simulink model "JC_20220328_1432"  (R2021a)
settings: Solver=FixedStepAuto  StartTime=0.0  StopTime=inf  FixedStep=1e-3  RelTol=1e-3  EnableMultiTasking=on
values from neighbouring files (symbols this model uses):
  a = 1.43208    [1DoFRollParam.mat]
  b = 1.62792    [1DoFRollParam.mat]    (also in cmenv_20220308_0532.m = ~isempty(strfind(computer, '64')))
  Cq = 8888.064375    [1DoFRollParam.mat]
  FzF_0_w = 6523.65    [1DoFRollParam.mat]
  FzR_0_w = 5738.85    [1DoFRollParam.mat]
  h_CoG = 0.642    [1DoFRollParam.mat]
  h_RC = 0.116    [1DoFRollParam.mat]
  hs = 0.526    [1DoFRollParam.mat]
  hu = 0.4    [1DoFRollParam.mat]
  Ix = 850    [1DoFRollParam.mat]
  Iz = 4600    [1DoFRollParam.mat]
  Kq = 138929.062472    [1DoFRollParam.mat]
  M = 2500    [1DoFRollParam.mat]
  M_damp_f = [-2800.47 -2055.7 -1627.71 -1221.625 -703.4875 0 703.4875 1221.625 1627.71 2055.7 2800.47]    [1DoFRollParam.mat]
  M_damp_r = [-2742.3 -2013 -1593.9 -1196.25 -688.875 0 688.875 1196.25 1593.9 2013 2742.3]    [1DoFRollParam.mat]
  Mf_stiff = [-6881.2026603 -6818.65169539 -6756.10058191 -6693.54932121 -6630.99791467 -6568.44636364 -6505.89466949 -6443.34283357 -6380.79085727 -6318.23874192 -6255.68648891 -6193.13409959 ... (221 elements, 1x221)]    [1DoFRollParam.mat]    (also in roll_stiffness.mat)
  Mr_stiff = [-8903.36440298 -8822.14706815 -8740.93733551 -8659.73513552 -8578.54039868 -8497.35305544 -8416.17303626 -8335.00027161 -8253.83469192 -8172.67622765 -8091.52480923 -8010.38036709 ... (221 elements, 1x221)]    [1DoFRollParam.mat]    (also in roll_stiffness.mat)
  ms = 2159    [1DoFRollParam.mat]
  mu = 341    [1DoFRollParam.mat]
  theta_dot_f_damp = [-0.617210682493 -0.308605341246 -0.154302670623 -0.0593471810089 -0.0237388724036 0 0.0237388724036 0.0593471810089 0.154302670623 0.308605341246 0.617210682493]    [1DoFRollParam.mat]
  theta_dot_r_damp = [-0.630303030303 -0.315151515152 -0.157575757576 -0.0606060606061 -0.0242424242424 0 0.0242424242424 0.0606060606061 0.157575757576 0.315151515152 0.630303030303]    [1DoFRollParam.mat]
  theta_f_stiff = [-0.13056379822 -0.129376854599 -0.128189910979 -0.127002967359 -0.125816023739 -0.124629080119 -0.123442136499 -0.122255192878 -0.121068249258 -0.119881305638 -0.118694362018 -0.117507418398 ... (221 elements, 1x221)]    [1DoFRollParam.mat]    (also in roll_stiffness.mat)
  theta_r_stiff = [-0.133333333333 -0.132121212121 -0.130909090909 -0.129696969697 -0.128484848485 -0.127272727273 -0.126060606061 -0.124848484848 -0.123636363636 -0.122424242424 -0.121212121212 -0.12 ... (221 elements, 1x221)]    [1DoFRollParam.mat]    (also in roll_stiffness.mat)
  tw = 1.6675    [1DoFRollParam.mat]
undefined symbols (not defined in the file or in its folder): Continuous, DiscIntNeverNeededParam, params, Time, X0
libraries: CarMaker4SL x52, simulink x2, ctrlSharedLib x2
(part 3 of 3)

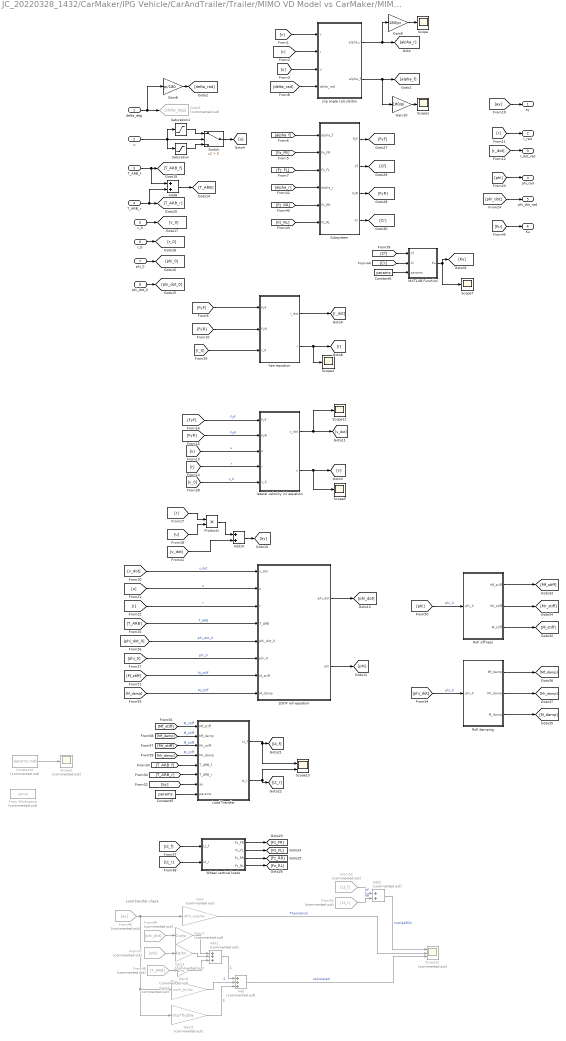
== system JC_20220328_1432/CarMaker/IPG Vehicle/CarAndTrailer/Trailer/MIMO VD Model vs CarMaker/MIMO 1DOF roll with LT1 ==
  note: Load transfer check
  delta_deg : Inport
  u : Inport  Port=2
  T_ARB_f : Inport  Port=3
  T_ARB_r : Inport  Port=4
  v_0 : Inport  Port=5
  r_0 : Inport  Port=6
  phi_0 : Inport  Port=7
  phi_dot_0 : Inport  Port=8
  1DOF roll equation : Subsystem
  Add : Sum  Commented=on  Inputs=+++
  Add1 : Sum  Commented=on  Inputs=+++
  Add10 : Sum
  Add2 : Sum  Commented=on
  Add8 : Sum
  Constant4 : Constant  Commented=on  Value=params.mat
  Constant5 : Constant  Value=params
  Constant6 : Constant  Value=params
  From Workspace : FromWorkspace  Commented=on  VariableName=simin
  From46 : From  Commented=on  GotoTag=ay
  From47 : From  Commented=on  GotoTag=phi
  From48 : From  Commented=on  GotoTag=T_ARB
  From49 : From  Commented=on  GotoTag=phi_dot
  From52 : From  Commented=on  GotoTag=Lt_f
  From53 : From  Commented=on  GotoTag=Lt_r
  Gain : Gain  Commented=on  Gain=M*h_CoG/tw
  Gain1 : Gain  Commented=on  Gain=Kq/tw
  Gain10 : Gain  Gain=180/pi
  Gain4 : Gain  Commented=on  Gain=ms*h_RC/tw
  Gain5 : Gain  Commented=on  Gain=mu*hu/tw
  Gain6 : Gain  Commented=on  Gain=1/tw
  Gain7 : Gain  Commented=on  Gain=Cq/tw
  Gain8 : Gain  Gain=pi/180
  Gain9 : Gain  Gain=180/pi
  Goto5 : Goto  Commented=on  GotoTag=delta_deg
  Load Transfer : MATLAB Function  TreatAsAtomicUnit=on
  MATLAB Function : MATLAB Function  TreatAsAtomicUnit=on
  Product1 : Product
  Roll damping : Subsystem
  Roll siffness : Subsystem
  Saturation : Saturate  UpperLimit=-eps  LowerLimit=-inf
  Saturation1 : Saturate  UpperLimit=inf  LowerLimit=eps
  Scope{,1,4..5,7,11} (6 alike) : Scope
  Scope12 : Scope  Commented=on  NumInputPorts=3
  Scope13 : Scope  NumInputPorts=2
  Scope2 : Scope  Commented=on
  Subsystem : Subsystem
      settings: AttributesFormatString=%<MinAlgLoopOccurrences>
  Switch : Switch  Criteria=u2 > Threshold
  Wheel vertical loads : Subsystem
      settings: AttributesFormatString=%<MinAlgLoopOccurrences>
  Yaw equation : Subsystem
  lateral velocity (v) equation : Subsystem
  slip angle calculaiton : Subsystem
  ay : Outport
  r_rad : Outport  Port=2
  r_dot_rad : Outport  Port=3
  phi_rad : Outport  Port=4
  phi_dot_rad : Outport  Port=5
  Ku : Outport  Port=6
  wires:
  delta_deg/1 -> Gain8/1, Goto5/1
  [r] -> r_rad/1
  [r_dot] -> r_dot_rad/1
  [r] -> Product1/1
  [u] -> Product1/2
  [ay] -> ay/1
  Gain8/1 -> [delta_rad]
  Gain10/1 -> Scope1/1
  Gain9/1 -> Scope/1
  [phi] -> phi_rad/1
  [phi_dot] -> phi_dot_rad/1
  phi_dot_0/1 -> [phi_dot_0]
  T_ARB_f/1 -> Add8/1, [T_ARB_f]
  T_ARB_r/1 -> Add8/2, [T_ARB_r]
  Add8/1 -> [T_ARB]
  [T_ARB_r] -> Load Transfer/6(T_ARB_r)
  [T_ARB_f] -> Load Transfer/5(T_ARB_f)
  Load Transfer/1(Lt_f) -> Scope13/1, [Lt_f]
  Load Transfer/2(Lt_r) -> Scope13/2, [Lt_r]
  Add10/1 -> [ay]
  Product1/1 -> Add10/1
  [v_dot] -> Add10/2
  [ay] -> Load Transfer/7(ay)
  [Lt_r] -> Wheel vertical loads/2(Lt_r)
  [Lt_f] -> Wheel vertical loads/1(Lt_f)
  Wheel vertical loads/1(Fz_FR) -> [Fz_FR]
  Wheel vertical loads/2(Fz_FL) -> [Fz_FL]
  Wheel vertical loads/3(Fz_RR) -> [Fz_RR]
  Wheel vertical loads/4(Fz_RL) -> [Fz_RL]
  slip angle calculaiton/2(alpha_f) -> Gain10/1, [alpha_f]
  slip angle calculaiton/1(alpha_r) -> [alpha_r], Gain9/1
  [v] -> slip angle calculaiton/1(v)
  [r] -> slip angle calculaiton/2(r)
  [u] -> slip angle calculaiton/3(u)
  [delta_rad] -> slip angle calculaiton/4(delta_rad)
  [alpha_f] -> Subsystem/1(alpha_f)
  [Fz_FR] -> Subsystem/2(Fz_FR)
  [Fz_FL] -> Subsystem/3(Fz_FL)
  [alpha_r] -> Subsystem/4(alpha_r)
  [Fz_RR] -> Subsystem/5(Fz_RR)
  [Fz_RL] -> Subsystem/6(Fz_RL)
  Subsystem/1(FyF) -> [FyF]
  Subsystem/3(FyR) -> [FyR]
  [Cr] -> MATLAB Function/2(Cr)
  [Cf] -> MATLAB Function/1(Cf)
  MATLAB Function/1(Ku) -> Scope7/1, [Ku]
  [Ku] -> Ku/1
  Subsystem/4(Cr) -> [Cr]
  Subsystem/2(Cf) -> [Cf]
  Yaw equation/2(r) -> [r], Scope4/1
  [FyF] -> Yaw equation/1(FyF)
  [FyR] -> Yaw equation/2(FyR)
  [r_0] -> Yaw equation/3(r_0)
  Yaw equation/1(r_dot) -> [r_dot]
  lateral velocity (v) equation/2(v) -> [v], Scope5/1
  lateral velocity (v) equation/1(v_dot) -> [v_dot], Scope11/1
  [FyF] -> lateral velocity (v) equation/1(FyF)  "FyF"
  [FyR] -> lateral velocity (v) equation/2(FyR)  "FyR"
  [u] -> lateral velocity (v) equation/3(u)  "u"
  [r] -> lateral velocity (v) equation/4(r)  "r"
  [v_0] -> lateral velocity (v) equation/5(v_0)  "v_0"
  [v_dot] -> 1DOF roll equation/1(v_dot)  "v_dot"
  [u] -> 1DOF roll equation/2(u)  "u"
  [r] -> 1DOF roll equation/3(r)  "r"
  [T_ARB] -> 1DOF roll equation/4(T_ARB)  "T_ARB"
  [phi_dot_0] -> 1DOF roll equation/5(phi_dot_0)  "phi_dot_0"
  [phi_0] -> 1DOF roll equation/6(phi_0)  "phi_0"
  1DOF roll equation/1(phi_dot) -> [phi_dot]
  1DOF roll equation/2(phi) -> [phi]
  phi_0/1 -> [phi_0]
  r_0/1 -> [r_0]
  v_0/1 -> [v_0]
  From46/1 -> Gain5/1, Gain4/1, Gain/1
  Gain/1 -> Scope12/2  "Theoretical"
  From47/1 -> Gain1/1
  Gain4/1 -> Add/2  "2"
  Gain5/1 -> Add/3  "3"
  Add/1 -> Scope12/3  "calculated"
  Gain1/1 -> Add1/2
  Add1/1 -> Add/1  "1"
  From48/1 -> Gain6/1
  Gain6/1 -> Add1/3
  From49/1 -> Gain7/1
  Gain7/1 -> Add1/1
  Add2/1 -> Scope12/1  "matlabFCN"
  From53/1 -> Add2/2  "ltR"
  From52/1 -> Add2/1  "ltF"
  [phi] -> Roll siffness/1(phi_0)  "phi_0"
  Roll siffness/1(Mf_stiff) -> [Mf_stiff]
  Roll siffness/3(M_stiff) -> [M_stiff]
  Roll siffness/2(Mr_stiff) -> [Mr_stiff]
  [M_stiff] -> 1DOF roll equation/7(M_stiff)  "M_stiff"
  Roll damping/3(M_damp) -> [M_damp]
  Roll damping/1(Mf_damp) -> [Mf_damp]
  Roll damping/2(Mr_damp) -> [Mr_damp]
  [phi_dot] -> Roll damping/1(phi_0)  "phi_0"
  [M_damp] -> 1DOF roll equation/8(M_damp)  "M_stiff"
  [Mf_stiff] -> Load Transfer/1(Mf_stiff)  "M_stiff"
  [Mf_damp] -> Load Transfer/2(Mf_damp)  "M_stiff"
  [Mr_stiff] -> Load Transfer/3(Mr_stiff)  "M_stiff"
  [Mr_damp] -> Load Transfer/4(Mr_damp)  "M_stiff"
  Constant4/1 -> Scope2/1
  Constant5/1 -> Load Transfer/8(params)
  Constant6/1 -> MATLAB Function/3(params)
  Saturation1/1 -> Switch/1
  u/1 -> Saturation/1, Saturation1/1, Switch/2
  Saturation/1 -> Switch/3
  Switch/1 -> [u]

== system JC_20220328_1432/CarMaker/IPG Vehicle/CarAndTrailer/Trailer/MIMO VD Model vs CarMaker/MIMO 1DOF roll with LT1/1DOF roll equation ==
  v_dot : Inport
  u : Inport  Port=2
  r : Inport  Port=3
  T_ARB : Inport  Port=4
  phi_dot_0 : Inport  Port=5
  phi_0 : Inport  Port=6
  M_stiff : Inport  Port=7
  M_damp : Inport  Port=8
  Add6 : Sum
  Add7 : Sum  Inputs=+---
  Gain11 : Gain  Gain=1/Ix
  Gain12 : Gain  Gain=ms*hs
  Integrator2 : Integrator  InitialConditionSource=external
  Integrator3 : Integrator  InitialConditionSource=external
  Product2 : Product
  phi_dot : Outport
  phi : Outport  Port=2
  wires:
  Gain11/1 -> Integrator2/1  "phi_dot_dot"
  Integrator3/1 -> phi/1  "phi"
  Integrator2/1 -> phi_dot/1, Integrator3/1  "phi_dot"
  Add7/1 -> Gain11/1
  Add6/1 -> Gain12/1
  Product2/1 -> Add6/2
  Gain12/1 -> Add7/1
  phi_0/1 -> Integrator3/2
  v_dot/1 -> Add6/1
  phi_dot_0/1 -> Integrator2/2
  T_ARB/1 -> Add7/4
  u/1 -> Product2/1
  r/1 -> Product2/2
  M_stiff/1 -> Add7/2
  M_damp/1 -> Add7/3

== system JC_20220328_1432/CarMaker/IPG Vehicle/CarAndTrailer/Trailer/MIMO VD Model vs CarMaker/MIMO 1DOF roll with LT1/Roll damping ==
  phi_0 : Inport
  Add3 : Sum
  Front roll damping : Lookup_n-D  NumberOfTableDimensions=1  BreakpointsForDimension1=theta_dot_f_damp  Table=M_damp_f  InternalRulePriority=Speed  RndMeth=Simplest  InputSameDT=on
  Rear roll damping : Lookup_n-D  NumberOfTableDimensions=1  BreakpointsForDimension1=theta_dot_r_damp  Table=M_damp_r  InternalRulePriority=Speed  RndMeth=Simplest  InputSameDT=on
  Mf_damp : Outport
  Mr_damp : Outport  Port=2
  M_damp : Outport  Port=3
  wires:
  Front roll damping/1 -> Mf_damp/1, Add3/1
  phi_0/1 -> Rear roll damping/1, Front roll damping/1
  Rear roll damping/1 -> Mr_damp/1, Add3/2
  Add3/1 -> M_damp/1

== system JC_20220328_1432/CarMaker/IPG Vehicle/CarAndTrailer/Trailer/MIMO VD Model vs CarMaker/MIMO 1DOF roll with LT1/Roll siffness ==
  phi_0 : Inport
  Add3 : Sum
  Front roll stiffness : Lookup_n-D  NumberOfTableDimensions=1  BreakpointsForDimension1=theta_f_stiff  Table=Mf_stiff  InternalRulePriority=Speed  RndMeth=Simplest  InputSameDT=on
  Rear roll stiffness : Lookup_n-D  NumberOfTableDimensions=1  BreakpointsForDimension1=theta_r_stiff  Table=Mr_stiff  InternalRulePriority=Speed  RndMeth=Simplest  InputSameDT=on
  Mf_stiff : Outport
  Mr_stiff : Outport  Port=2
  M_stiff : Outport  Port=3
  wires:
  Front roll stiffness/1 -> Mf_stiff/1, Add3/1
  phi_0/1 -> Rear roll stiffness/1, Front roll stiffness/1
  Rear roll stiffness/1 -> Mr_stiff/1, Add3/2
  Add3/1 -> M_stiff/1

== system JC_20220328_1432/CarMaker/IPG Vehicle/CarAndTrailer/Trailer/MIMO VD Model vs CarMaker/MIMO 1DOF roll with LT1/Subsystem ==
  alpha_f : Inport
  Fz_FR : Inport  Port=2
  Fz_FL : Inport  Port=3
  alpha_r : Inport  Port=4
  Fz_RR : Inport  Port=5
  Fz_RL : Inport  Port=6
  Add{,1..3} (4 alike) : Sum
  Front tire formula : MATLAB Function  TreatAsAtomicUnit=on
      settings: AttributesFormatString=%<MinAlgLoopOccurrences>  MinAlgLoopOccurrences=on
  Front tire formula1 : MATLAB Function  TreatAsAtomicUnit=on
      settings: MinAlgLoopOccurrences=on
  Rear tire formula : MATLAB Function  TreatAsAtomicUnit=on
      settings: MinAlgLoopOccurrences=on
  Rear tire formula1 : MATLAB Function  TreatAsAtomicUnit=on
      settings: MinAlgLoopOccurrences=on
  Scope1 : Scope  NumInputPorts=2
  FyF : Outport
  Cf : Outport  Port=2
  FyR : Outport  Port=3
  Cr : Outport  Port=4
  wires:
  Rear tire formula/1(Fy) -> Add1/1  "FyRR"
  Fz_RL/1 -> Rear tire formula1/2(Fz)
  Fz_RR/1 -> Rear tire formula/2(Fz)
  Rear tire formula1/1(Fy) -> Add1/2  "FyRL"
  Fz_FR/1 -> Front tire formula/2(Fz)
  Fz_FL/1 -> Front tire formula1/2(Fz)
  alpha_f/1 -> Front tire formula1/1(alpha_f), Front tire formula/1(alpha_f)
  alpha_r/1 -> Rear tire formula1/1(alpha_r), Rear tire formula/1(alpha_r)
  Front tire formula/1(Fy) -> Scope1/1, Add/1  "FyFR"
  Front tire formula1/1(Fy) -> Scope1/2, Add/2  "FYFL"
  Add/1 -> FyF/1
  Add1/1 -> FyR/1
  Front tire formula/2(C_f) -> Add2/1
  Front tire formula1/2(C_f) -> Add2/2
  Add2/1 -> Cf/1
  Rear tire formula/2(C_r) -> Add3/1
  Rear tire formula1/2(C_r) -> Add3/2
  Add3/1 -> Cr/1

== system JC_20220328_1432/CarMaker/IPG Vehicle/CarAndTrailer/Trailer/MIMO VD Model vs CarMaker/MIMO 1DOF roll with LT1/Wheel vertical loads ==
  Lt_f : Inport
  Lt_r : Inport  Port=2
  Constant : Constant  Value=FzF_0_w
  Constant1 : Constant  Value=FzR_0_w
  Sum : Sum  Inputs=|++
  Sum1 : Sum  Inputs=|++
  Sum2 : Sum  Inputs=+-|
  Sum3 : Sum  Inputs=+-|
  Fz_FR : Outport
  Fz_FL : Outport  Port=2
  Fz_RR : Outport  Port=3
  Fz_RL : Outport  Port=4
  wires:
  Constant/1 -> Sum2/1, Sum/1
  Constant1/1 -> Sum1/1, Sum3/1
  Sum1/1 -> Fz_RR/1
  Lt_f/1 -> Sum/2, Sum2/2
  Sum/1 -> Fz_FR/1
  Sum2/1 -> Fz_FL/1
  Lt_r/1 -> Sum1/2, Sum3/2
  Sum3/1 -> Fz_RL/1

== system JC_20220328_1432/CarMaker/IPG Vehicle/CarAndTrailer/Trailer/MIMO VD Model vs CarMaker/MIMO 1DOF roll with LT1/Yaw equation ==
  FyF : Inport
  FyR : Inport  Port=2
  r_0 : Inport  Port=3
  Add3 : Sum  Inputs=+-
  Gain4 : Gain  Gain=1/Iz
  Gain5 : Gain  Gain=a
  Gain6 : Gain  Gain=b
  Integrator : Integrator  InitialConditionSource=external
  r_dot : Outport
  r : Outport  Port=2
  wires:
  Gain4/1 -> r_dot/1, Integrator/1  "r_dot"
  FyF/1 -> Gain5/1
  r_0/1 -> Integrator/2
  Gain5/1 -> Add3/1
  Gain6/1 -> Add3/2
  Add3/1 -> Gain4/1
  FyR/1 -> Gain6/1
  Integrator/1 -> r/1  "r"

== system JC_20220328_1432/CarMaker/IPG Vehicle/CarAndTrailer/Trailer/MIMO VD Model vs CarMaker/MIMO 1DOF roll with LT1/lateral velocity (v) equation ==
  FyF : Inport
  FyR : Inport  Port=2
  u : Inport  Port=3
  r : Inport  Port=4
  v_0 : Inport  Port=5
  Add4 : Sum  Inputs=+-
  Add5 : Sum
  Gain7 : Gain  Gain=1/M
  Integrator1 : Integrator  InitialConditionSource=external
  Product : Product
  v_dot : Outport
  v : Outport  Port=2
  wires:
  Add4/1 -> v_dot/1, Integrator1/1  "v_dot"
  FyF/1 -> Add5/1
  Product/1 -> Add4/2
  Gain7/1 -> Add4/1
  Add5/1 -> Gain7/1
  Integrator1/1 -> v/1  "v"
  r/1 -> Product/2
  u/1 -> Product/1
  FyR/1 -> Add5/2
  v_0/1 -> Integrator1/2

== system JC_20220328_1432/CarMaker/IPG Vehicle/CarAndTrailer/Trailer/MIMO VD Model vs CarMaker/MIMO 1DOF roll with LT1/slip angle calculaiton ==
  v : Inport
  r : Inport  Port=2
  u : Inport  Port=3
  delta_rad : Inport  Port=4
  Add : Sum  Inputs=-+
  Add1 : Sum
  Add2 : Sum  Inputs=+-
  Divide : Product  Inputs=*/
  Divide1 : Product  Inputs=*/
  Gain : Gain  Gain=b
  Gain1 : Gain  Gain=a
  alpha_r : Outport
  alpha_f : Outport  Port=2
  wires:
  Gain1/1 -> Add1/2
  Divide1/1 -> Add2/2
  Add/1 -> Divide/1
  Add1/1 -> Divide1/1
  delta_rad/1 -> Add2/1
  r/1 -> Gain1/1, Gain/1
  Gain/1 -> Add/2
  Add2/1 -> alpha_f/1
  v/1 -> Add1/1, Add/1
  Divide/1 -> alpha_r/1
  u/1 -> Divide1/2, Divide/2

== matlab function JC_20220328_1432/CarMaker/IPG Vehicle/CarAndTrailer/Trailer/MIMO VD Model vs CarMaker/MIMO 1DOF roll with LT1/Load Transfer ==
  data: Mf_stiff input; Mf_damp input; Mr_stiff input; Mr_damp input; Lt_f output; Lt_r output; T_ARB_f input; T_ARB_r input; ay input; params input
function [Lt_f, Lt_r] = fcn(Mf_stiff, Mf_damp, Mr_stiff, Mr_damp, T_ARB_f, T_ARB_r, ay, params)

mu_f = params(1);
mu_r = params(2);
ms_f = params(3);
ms_r = params(4);
hu = params(5);
h_RC = params(6);
tw_F = params(7);
tw_R = params(8);

% St = load('params.mat');
% St2 = load('params2.mat');


%% Load transfer in the front
Ltf_1 = (Mf_stiff + Mf_damp + T_ARB_f)/tw_F; %% Load transfer due to roll (front)
Ltf_2 = ms_f*ay*h_RC/tw_F;
Ltf_3 = mu_f*ay*hu/tw_F;

Lt_f = Ltf_1 + Ltf_2 + Ltf_3;

%% Load transfer in the rear
Ltr_1 = (Mr_stiff + Mr_damp + T_ARB_r)/tw_R; %% Load transfer due to roll (front)
Ltr_2 = ms_r*ay*h_RC/tw_R;
Ltr_3 = mu_r*ay*hu/tw_R;

Lt_r = Ltr_1 + Ltr_2 + Ltr_3;

== matlab function JC_20220328_1432/CarMaker/IPG Vehicle/CarAndTrailer/Trailer/MIMO VD Model vs CarMaker/MIMO 1DOF roll with LT1/MATLAB Function ==
  data: Cf input; Ku output; Cr input; params input
function Ku = fcn(Cf, Cr, params)

a = params(9);
b = params(10);
M = params(11);
L = params(12);


Ku = M/L*((b*Cr - a*Cf)/(Cf*Cr));

== matlab function JC_20220328_1432/CarMaker/IPG Vehicle/CarAndTrailer/Trailer/MIMO VD Model vs CarMaker/MIMO 1DOF roll with LT1/Subsystem/Front tire formula ==
  data: alpha_f input; Fy output; Fz input; C_f output
function [Fy, C_f] = fcn(alpha_f, Fz)
%% Pajecka formula for the front axle

mu_peak = 1.37 - Fz*0.026/1000;
mu_90_deg_f = 0.723*mu_peak;

Bf = 13; %% stiffness factor. Gives maximum mu for alpha = 6º for the static front tyre load.
Cf = 1.515; % Makes mu_max/mu_90_deg=0.723 for static front tyre load
Df = mu_peak; %% peak value. If Df<Dr understeer
Ef = Fz*(0.5+2)/12000 - 2; %% Curvature factor. Linear variation from Fz = 0KN to 12KN

mu_y_f = Df.*sin(Cf.*atan(Bf*alpha_f - Ef*(Bf*alpha_f - atan(Bf*alpha_f))));

n_f = (Cf.*Df.*cos(Cf.*atan(Bf.*alpha_f + Ef.*(atan(Bf.*alpha_f) - Bf.*alpha_f))).*(Bf - Ef.*(Bf - Bf./(Bf.^2.*alpha_f.^2 + 1))))./((Bf.*alpha_f + Ef.*(atan(Bf.*alpha_f) - Bf.*alpha_f)).^2 + 1);
C_f = n_f.*Fz;

Fy = mu_y_f*Fz;

% Fy = alpha;

== matlab function JC_20220328_1432/CarMaker/IPG Vehicle/CarAndTrailer/Trailer/MIMO VD Model vs CarMaker/MIMO 1DOF roll with LT1/Subsystem/Front tire formula1 ==
  data: alpha_f input; Fy output; Fz input; C_f output
function [Fy, C_f] = fcn(alpha_f, Fz)
%% Pajecka formula for the front axle

mu_peak = 1.37 - Fz*0.026/1000;
mu_90_deg_f = 0.723*mu_peak;

Bf = 13; %% stiffness factor. Gives maximum mu for alpha = 6º for the static front tyre load.
Cf = 1.515; % Makes mu_max/mu_90_deg=0.723 for static front tyre load
Df = mu_peak; %% peak value. If Df<Dr understeer
Ef = Fz*(0.5+2)/12000 - 2; %% Curvature factor. Linear variation from Fz = 0KN to 12KN

mu_y_f = Df.*sin(Cf.*atan(Bf*alpha_f - Ef*(Bf*alpha_f - atan(Bf*alpha_f))));

n_f = (Cf.*Df.*cos(Cf.*atan(Bf.*alpha_f + Ef.*(atan(Bf.*alpha_f) - Bf.*alpha_f))).*(Bf - Ef.*(Bf - Bf./(Bf.^2.*alpha_f.^2 + 1))))./((Bf.*alpha_f + Ef.*(atan(Bf.*alpha_f) - Bf.*alpha_f)).^2 + 1);
C_f = n_f.*Fz;

Fy = mu_y_f*Fz;

% Fy = alpha;

== matlab function JC_20220328_1432/CarMaker/IPG Vehicle/CarAndTrailer/Trailer/MIMO VD Model vs CarMaker/MIMO 1DOF roll with LT1/Subsystem/Rear tire formula ==
  data: alpha_r input; Fy output; Fz input; C_r output
function [Fy, C_r] = fcn(alpha_r, Fz)
%% Pajecka formula for the front axle

mu_peak_r = 1.38 - Fz*0.0232/1000;
mu_90_deg_r = 0.723*mu_peak_r;

Br = 13; %% stiffness factor. Gives maximum mu for alpha = 6º for the static front tyre load.
Cr = 1.51253; % Makes mu_max/mu_90_deg=0.723 for static front tyre load
Dr = mu_peak_r; %% peak value. If Df<Dr understeer
Er = Fz*(0.5+2)/12000 - 2; %% Curvature factor. Linear variation from Fz = 0KN to 12KN

mu_y_r = Dr.*sin(Cr.*atan(Br*alpha_r - Er*(Br*alpha_r - atan(Br*alpha_r))));
n_r = (Cr.*Dr.*cos(Cr.*atan(Br.*alpha_r + Er.*(atan(Br.*alpha_r) - Br.*alpha_r))).*(Br - Er.*(Br - Br./(Br.^2.*alpha_r.^2 + 1))))./((Br.*alpha_r + Er.*(atan(Br.*alpha_r) - Br.*alpha_r)).^2 + 1);
C_r = n_r.*Fz;

Fy = mu_y_r*Fz;

% Fy = alpha;

== matlab function JC_20220328_1432/CarMaker/IPG Vehicle/CarAndTrailer/Trailer/MIMO VD Model vs CarMaker/MIMO 1DOF roll with LT1/Subsystem/Rear tire formula1 ==
  data: alpha_r input; Fy output; Fz input; C_r output
function [Fy, C_r] = fcn(alpha_r, Fz)
%% Pajecka formula for the front axle

mu_peak_r = 1.38 - Fz*0.0232/1000;
mu_90_deg_r = 0.723*mu_peak_r;

Br = 13; %% stiffness factor. Gives maximum mu for alpha = 6º for the static front tyre load.
Cr = 1.51253; % Makes mu_max/mu_90_deg=0.723 for static front tyre load
Dr = mu_peak_r; %% peak value. If Df<Dr understeer
Er = Fz*(0.5+2)/12000 - 2; %% Curvature factor. Linear variation from Fz = 0KN to 12KN

mu_y_r = Dr.*sin(Cr.*atan(Br*alpha_r - Er*(Br*alpha_r - atan(Br*alpha_r))));
n_r = (Cr.*Dr.*cos(Cr.*atan(Br.*alpha_r + Er.*(atan(Br.*alpha_r) - Br.*alpha_r))).*(Br - Er.*(Br - Br./(Br.^2.*alpha_r.^2 + 1))))./((Br.*alpha_r + Er.*(atan(Br.*alpha_r) - Br.*alpha_r)).^2 + 1);
C_r = n_r.*Fz;

Fy = mu_y_r*Fz;

% Fy = alpha;
